simulink model "main"  (R2020a)
settings: Solver=FixedStepDiscrete  StartTime=0.0  StopTime=10.0  RelTol=1e-3
InitFcn:
  | mbd_s32k_consistency_checks(bdroot(gcs));
undefined symbols (not defined in the file or in its folder): LQFP
libraries: sldrtlib x13, simulink x6, mbd_s32k1xx_ec_toolbox x1
settings Model: Creator=ecs  LastModifiedBy=ecs
settings DataIOCC: ExternalInput=off  InitialState=off  SaveOutput=off  SignalLogging=off  SaveTime=off
settings OptimizationCC: DefaultParameterBehavior=Inlined  EnhancedBackFolding=on  PassReuseOutputArgsAs=Individual arguments  ZeroExternalMemoryAtStartup=off  ZeroInternalMemoryAtStartup=off  OptimizeBlockOrder=speed  DifferentSizesBufferReuse=on  OptimizationCustomize=off  EfficientTunableParamExpr=on
settings DebuggingCC: InheritedTsInSrcMsg=none  SingleTaskRateTransMsg=error  ParameterTunabilityLossMsg=error  UnconnectedInputMsg=error  UnconnectedOutputMsg=error  UnconnectedLineMsg=error  UnknownTsInhSupMsg=error
settings HardwareCC: ProdBitPerPointer=32  ProdBitPerSizeT=32  ProdBitPerPtrDiffT=32  ProdLargestAtomicInteger=Long  ProdLargestAtomicFloat=Double  ProdWordSize=32  ProdHWDeviceType=ARM Compatible->ARM Cortex
settings SFSimCC: MATLABDynamicMemAlloc=off
settings RTWCC: Description=Model Based Design Toolbox S32K1xx Code Generation Target  SystemTargetFile=mbd_s32k.tlc  MakeCommand=mbd_s32k_make_rtw COPY_MDLREF_INCLUDES=0  TemplateMakefile=mbd_s32k.tmf  GenerateReport=on  IncludeHyperlinkInReport=on  LaunchReport=on  GenerateTraceInfo=on  GenerateTraceReport=on  GenerateTraceReportSl=on  GenerateTraceReportSf=on  GenerateTraceReportEml=on  GenerateCodeMetricsReport=on
settings CodeAppCC: ForceParamTrailComments=on  IgnoreCustomStorageClasses=off  OperatorAnnotations=on  SimulinkDataObjDesc=on  SFDataObjDesc=on  InsertBlockDesc=on
settings STFCustomTargetCC: TargetLangStandard=C99 (ISO)  MultiwordLength=256  GenerateSampleERTMain=on  CombineOutputUpdateFcns=on  ERTCustomFileBanners=on  SupportContinuousTime=off  SupportNonInlinedSFcns=off  RemoveResetFunc=on  MATLABClassNameForMDSCustomization=Simulink.SoftwareTarget.ERTCustomization  SystemTargetFile=mbd_s32k.tlc
settings ERTTargetCC: TargetLangStandard=C99 (ISO)  GenerateSampleERTMain=on  ParMdlRefBuildCompliant=off  CompOptLevelCompliant=off  ConcurrentExecutionCompliant=off  ModelStepFunctionPrototypeControlCompliant=off  CPPClassGenCompliant=off  UseToolchainInfoCompliant=off  InlinedParameterPlacement=NonHierarchical  ERTSrcFileBannerTemplate=mbd_ert_code_template.cgt  ERTHdrFileBannerTemplate=mbd_ert_code_template.cgt  ERTDataSrcFileTemplate=mbd_ert_code_template.cgt  ERTDataHdrFileTemplate=mbd_ert_code_template.cgt  ERTCustomFileTemplate=example_file_process.tlc

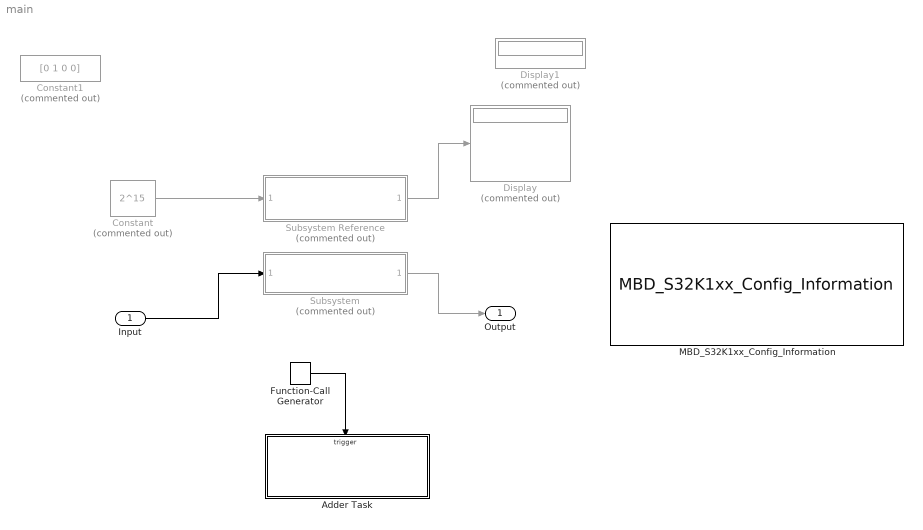
== system main ==
  Input : Inport
  Adder Task : Subsystem
  Constant : Constant  Commented=on  Value=2^15  OutDataTypeStr=uint32
  Constant1 : Constant  Commented=on  Value=[0 1 0 0]  OutDataTypeStr=uint8
  Display : Display  Commented=on
  Display1 : Display  Commented=on
  Function-Call Generator : simulink/Ports & Subsystems/Function-Call Generator  sample_time=0.1  numberOfIterations=1
  MBD_S32K1xx_Config_Information : mbd_s32k1xx_ec_toolbox/MBD_S32K1xx_Config_Information  mbdt_ver=0  disp_str=|  config_params=[]  mcu_target_name=S32K144  mcu_target_package=100-LQFP  mcu_target_sram_size=48KB  mcu_system_clock_freq=80  mcu_xtal_freq=External 8  mcu_steptick_timer=LPIT Channel 0  mcu_steptick_prio=15  ds_import_enable=on  target_compiler=GCC  target_memory=FLASH  gcc_target_compile_opts=-mthumb -mfloat-abi=hard -mfpu=fpv4-sp-d16 -O1 -g -gstrict-dwarf  gcc_target_assemble_opts=-mthumb -mfloat-abi=hard -mfpu=fpv4-sp-d16 -g  gcc_target_link_opts=-mthumb -mfloat-abi=hard -mfpu=fpv4-sp-d16  gcc_target_default_lcf=on  gcc_target_user_lcf=S32K148_192_flash.ld  ghs_target_compile_opts=-cpu=cortexm4f -thumb -fpu=vfpv4_d16 -fsingle -Ogeneral -Wundef -Wimplicit-int -Wshadow -Wtrigraphs --no_commons --gnu_asm -gnu99 -gdwarf-2 -G  ghs_target_assemble_opts=-cpu=cortexm4f -fpu=vfpv4_d16  ghs_target_link_opts=-cpu=cortexm4f -thumb -fpu=vfpv4_d16  ghs_target_default_lcf=on  ghs_target_user_lcf=S32K148_192_flash.ld  iar_target_compile_opts=--cpu=Cortex-M4F --thumb --fpu=VFPv4_sp -Ol -e --debug --dlib_config normal  iar_target_assemble_opts=--cpu Cortex-M4F --thumb --fpu VFPv4_sp  iar_target_link_opts=--no_exceptions --vfe --inline  iar_target_default_lcf=on  iar_target_user_lcf=S32K148_192_flash.icf  pil_download_enable=off  rbl_download_enable=on  rbl_start_delay=5000  rbl_download_interface=OpenSDA  rbl_restart_request=off  rbl_com_port=Custom  rbl_com_port_custom=COM1  pil_download_rate=57600  pil_opensda_drive=F: EVB-S32K144  pil_opensda_drive_custom=D  pil_uart_instance=1  pil_uart_rx=PTC6: [LPUART1_RX | Receive]  pil_uart_tx=PTC7: [LPUART1_TX | Transmit]  FTM_PWM_PcrCheckEnDis=on  FTM_Input_Edge_Inputs_PcrCheckEnDis=on  FTM_Dual_Edge_Inputs_PcrCheckEnDis=on  FTM_Quadrature_Inputs_PcrCheckEnDis=on  FTM_Hall_Sensor_Inputs_PcrCheckEnDis=on  LPTMR_PcrCheckEnDis=on  PIT_PcrCheckEnDis=on  RTC_PcrCheckEnDis=on  FlexCAN_PcrCheckEnDis=on  LIN_PcrCheckEnDis=on  FlexIO_PcrCheckEnDis=on  LPI2C_PcrCheckEnDis=on  LPSPI_PcrCheckEnDis=on  LPUART_PcrCheckEnDis=on  CMP_PcrCheckEnDis=on  GPIO_OutputPcrCheckEnDis=on  GPIO_InputPcrCheckEnDis=on  SBC_PcrCheckEnDis=on  AMMCLIB_PcrCheckEnDis=on  FM_PcrCheckEnDis=on  Profile_PcrCheckEnDis=on  ConfigParams_PcrCheckEnDis=on  ModelRef_PcrCheckEnDis=on  PDB0_PcrCheckEnDis=on  CSEc_PcrCheckEnDis=on  eDMA_PcrCheckEnDis=on  ADC_PcrCheckEnDis=on  WDOG_PcrCheckEnDis=on
      | Target : S32K144-64KB_SRAM
      | Package : 100-pin
      | System clock : 80 MHz
      | XTAL clock : External 8 MHz
      | Compiler : IAR
      | Target Type : FLASH
      | Download Code after build : off
      | Step Tick Interrupt Priority : 15
  Subsystem : Subsystem  Commented=on  ReferencedSubsystem=sub2
  Subsystem Reference : Subsystem  Commented=on  ReferencedSubsystem=sub1
  Output : Outport
  wires:
  Subsystem Reference/1 -> Display/1
  Constant/1 -> Subsystem Reference/1
  Input/1 -> Subsystem/1
  Subsystem/1 -> Output/1
  Function-Call Generator/1 -> Adder Task/Trigger

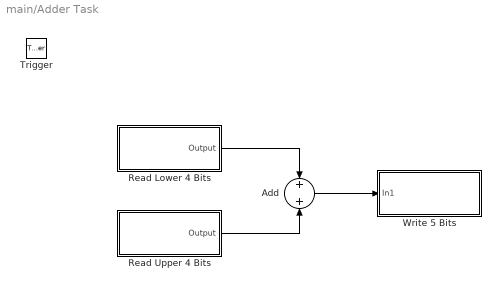
== system main/Adder Task ==
  Trigger : TriggerPort  TriggerType=function-call  VariantControl=Variant  PortDimensions=1
  Add : Sum
  Read Lower 4 Bits : Subsystem
  Read Upper 4 Bits : Subsystem
  Write 5 Bits : Subsystem
  wires:
  Read Lower 4 Bits/1(Output) -> Add/1
  Add/1 -> Write 5 Bits/1(In1)
  Read Upper 4 Bits/1(Output) -> Add/2

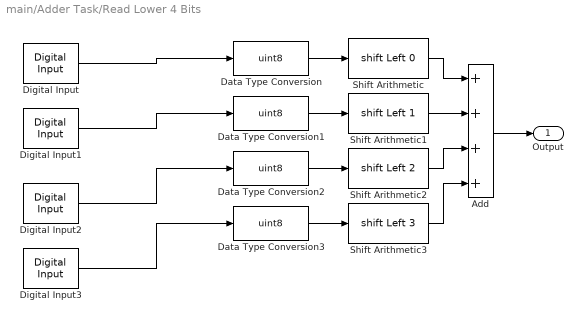
== system main/Adder Task/Read Lower 4 Bits ==
  Add : Sum  Inputs=++++
  Data Type Conversion{,1..3} (4 alike) : DataTypeConversion  OutDataTypeStr=uint8
  Digital Input{,1..3} (4 alike) : sldrtlib/Digital Input  SampleTime=0.1  MaxMissedTicks=10  ShowMissedTicks=off  YieldWhenWaiting=off  DrvAddress=0  DrvOptions=0  Channels=1  BitMode=1  DataType=1
      settings: SourceProductBaseCode=WT
  Shift Arithmetic : ArithShift  BitShiftDirection=Left
  Shift Arithmetic1 : ArithShift  BitShiftNumber=1  BitShiftDirection=Left
  Shift Arithmetic2 : ArithShift  BitShiftNumber=2  BitShiftDirection=Left
  Shift Arithmetic3 : ArithShift  BitShiftNumber=3  BitShiftDirection=Left
  Output : Outport  OutDataTypeStr=uint8
  wires:
  Data Type Conversion1/1 -> Shift Arithmetic1/1
  Shift Arithmetic3/1 -> Add/4
  Add/1 -> Output/1
  Data Type Conversion3/1 -> Shift Arithmetic3/1
  Data Type Conversion2/1 -> Shift Arithmetic2/1
  Shift Arithmetic/1 -> Add/1
  Data Type Conversion/1 -> Shift Arithmetic/1
  Shift Arithmetic1/1 -> Add/2
  Shift Arithmetic2/1 -> Add/3
  Digital Input1/1 -> Data Type Conversion1/1
  Digital Input2/1 -> Data Type Conversion2/1
  Digital Input3/1 -> Data Type Conversion3/1
  Digital Input/1 -> Data Type Conversion/1

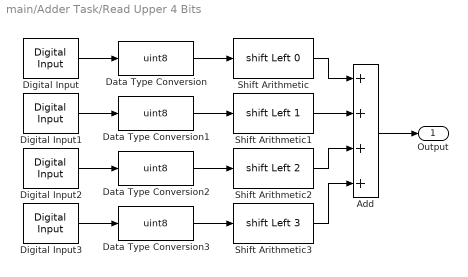
== system main/Adder Task/Read Upper 4 Bits ==
  Add : Sum  Inputs=++++
  Data Type Conversion{,1..3} (4 alike) : DataTypeConversion  OutDataTypeStr=uint8
  Digital Input{,1..3} (4 alike) : sldrtlib/Digital Input  SampleTime=0.1  MaxMissedTicks=10  ShowMissedTicks=off  YieldWhenWaiting=off  DrvAddress=0  DrvOptions=0  Channels=1  BitMode=1  DataType=1
      settings: SourceProductBaseCode=WT
  Shift Arithmetic : ArithShift  BitShiftDirection=Left
  Shift Arithmetic1 : ArithShift  BitShiftNumber=1  BitShiftDirection=Left
  Shift Arithmetic2 : ArithShift  BitShiftNumber=2  BitShiftDirection=Left
  Shift Arithmetic3 : ArithShift  BitShiftNumber=3  BitShiftDirection=Left
  Output : Outport  OutDataTypeStr=uint8
  wires:
  Data Type Conversion1/1 -> Shift Arithmetic1/1
  Shift Arithmetic3/1 -> Add/4
  Add/1 -> Output/1
  Data Type Conversion3/1 -> Shift Arithmetic3/1
  Data Type Conversion2/1 -> Shift Arithmetic2/1
  Shift Arithmetic/1 -> Add/1
  Data Type Conversion/1 -> Shift Arithmetic/1
  Shift Arithmetic1/1 -> Add/2
  Shift Arithmetic2/1 -> Add/3
  Digital Input1/1 -> Data Type Conversion1/1
  Digital Input2/1 -> Data Type Conversion2/1
  Digital Input3/1 -> Data Type Conversion3/1
  Digital Input/1 -> Data Type Conversion/1

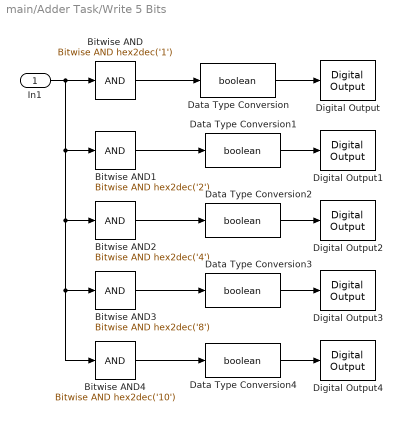
== system main/Adder Task/Write 5 Bits ==
  In1 : Inport  OutDataTypeStr=uint8
  Bitwise AND : simulink/Logic and Bit Operations/Bitwise Operator  logicop=AND  UseBitMask=on  BitMask=hex2dec('1')  BitMaskRealWorld=Stored Integer
  Bitwise AND1 : simulink/Logic and Bit Operations/Bitwise Operator  logicop=AND  UseBitMask=on  BitMask=hex2dec('2')  BitMaskRealWorld=Stored Integer
  Bitwise AND2 : simulink/Logic and Bit Operations/Bitwise Operator  logicop=AND  UseBitMask=on  BitMask=hex2dec('4')  BitMaskRealWorld=Stored Integer
  Bitwise AND3 : simulink/Logic and Bit Operations/Bitwise Operator  logicop=AND  UseBitMask=on  BitMask=hex2dec('8')  BitMaskRealWorld=Stored Integer
  Bitwise AND4 : simulink/Logic and Bit Operations/Bitwise Operator  logicop=AND  UseBitMask=on  BitMask=hex2dec('10')  BitMaskRealWorld=Stored Integer
  Data Type Conversion{,1..4} (5 alike) : DataTypeConversion  OutDataTypeStr=boolean
  Digital Output{,1..4} (5 alike) : sldrtlib/Digital Output  SampleTime=0.1  MaxMissedTicks=10  ShowMissedTicks=off  YieldWhenWaiting=off  DrvAddress=0  DrvOptions=0  Channels=1  BitMode=1  InitialValue=[]  FinalValue=[]
      settings: SourceProductBaseCode=WT
  wires:
  Bitwise AND1/1 -> Data Type Conversion1/1
  Bitwise AND4/1 -> Data Type Conversion4/1
  Data Type Conversion2/1 -> Digital Output2/1
  Data Type Conversion4/1 -> Digital Output4/1
  Bitwise AND3/1 -> Data Type Conversion3/1
  Bitwise AND/1 -> Data Type Conversion/1
  Bitwise AND2/1 -> Data Type Conversion2/1
  Data Type Conversion1/1 -> Digital Output1/1
  Data Type Conversion/1 -> Digital Output/1
  Data Type Conversion3/1 -> Digital Output3/1
  In1/1 -> Bitwise AND4/1, Bitwise AND3/1, Bitwise AND2/1, Bitwise AND1/1, Bitwise AND/1
